simulink model "TransferFunction"  (R2024b)
settings: Solver=VariableStepAuto  StartTime=0.0  StopTime=20  RelTol=1e-3
settings Model: Creator=bolinsfe  LastModifiedBy=bolinsfe

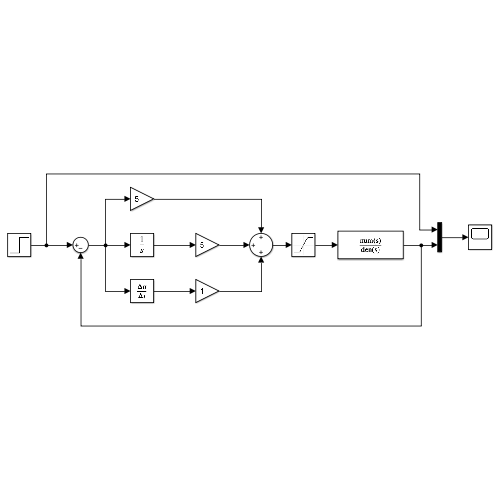
[thumbnail: Simulink's stored preview of the top-level diagram]
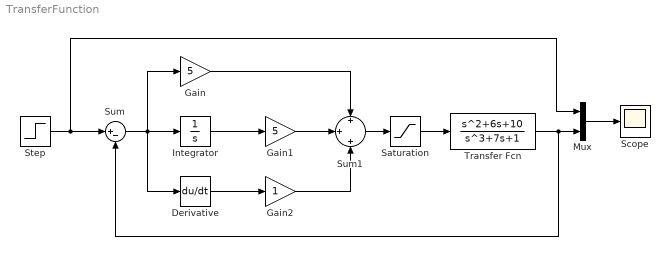
== system TransferFunction ==
  Derivative : Derivative
  Gain : Gain  Gain=5
  Gain1 : Gain  Gain=5
  Gain2 : Gain
  Integrator : Integrator
  Mux : Mux  Inputs=2
  Saturation : Saturate
  Scope : Scope
  Step : Step  SampleTime=0
  Sum : Sum  Inputs=|+-
  Sum1 : Sum  Inputs=+|+|+
  Transfer Fcn : TransferFcn  Numerator=[1 6 10]  Denominator=[1 0 7 1]
  wires:
  Step/1 -> Mux/1, Sum/1
  Transfer Fcn/1 -> Mux/2, Sum/2
  Integrator/1 -> Gain1/1
  Sum/1 -> Derivative/1, Integrator/1, Gain/1
  Gain/1 -> Sum1/1
  Mux/1 -> Scope/1
  Sum1/1 -> Saturation/1
  Derivative/1 -> Gain2/1
  Gain1/1 -> Sum1/2
  Gain2/1 -> Sum1/3
  Saturation/1 -> Transfer Fcn/1
